simulink model "FSK_switched"  (R2019a)
settings: Solver=ode45  StartTime=0.0  StopTime=10.0  RelTol=1e-3  EnableMultiTasking=on
libraries: commnoisgen2 x1, dspobslib x1
settings Model: Creator=carlos  LastModifiedBy=carlos
settings DataIOCC: LimitDataPoints=on  SaveFormat=Array  SignalLoggingSaveFormat=ModelDataLogs  ReturnWorkspaceOutputs=off
settings OptimizationCC: ExpressionDepthLimit=2147483647  LifeSpan=inf
settings DebuggingCC: UnderspecifiedInitializationDetection=Classic  MergeDetectMultiDrivingBlocksExec=none  SolverPrmCheckMsg=warning  FcnCallInpInsideContextMsg=warning  StateNameClashWarn=warning  SFUnexpectedBacktrackingDiag=warning  SFNoUnconditionalDefaultTransitionDiag=warning  SFExecutionAtInitializationDiag=none  ArithmeticOperatorsInVariantConditions=warning
settings HardwareCC: ProdBitPerPointer=32  ProdBitPerSizeT=32  ProdBitPerPtrDiffT=32  ProdLargestAtomicFloat=None  ProdIntDivRoundTo=Undefined  ProdEndianess=Unspecified  ProdWordSize=32  ProdHWDeviceType=32-bit Generic
settings ModelReferenceCC: PropagateSignalLabelsOutOfModel=off
settings SFSimCC: SimUseLocalCustomCode=off
settings RTWCC: RTWUseLocalCustomCode=off
settings CodeAppCC: StateflowObjectComments=on
settings GRTTargetCC: TargetLangStandard=C89/C90 (ANSI)  CombineOutputUpdateFcns=off  GRTInterface=on
settings ConfigComp: CovMetricSettings=dw  CovHtmlReporting=on  CovSaveCumulativeToWorkspaceVar=on  CovSaveSingleToWorkspaceVar=on  CovExternalEMLEnable=off

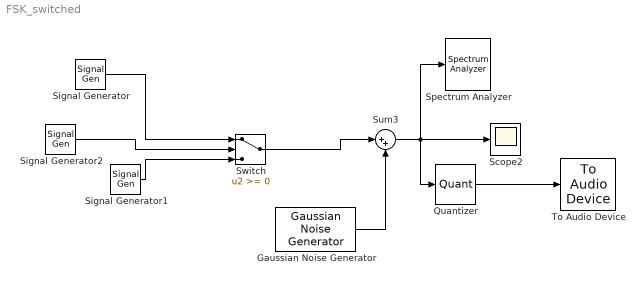
== system FSK_switched ==
  Gaussian Noise Generator : commnoisgen2/Gaussian Noise Generator  m=0  d=0  s=200  Ts=1e-4  frameBased=off  sampPerFrame=1  orient=off  outDataType=double
      settings: SourceProductName=Communications Toolbox  SourceProductBaseCode=CM
  Quantizer : Quantizer  QuantizationInterval=0.01  LinearizeAsGain=off  SampleTime=1/44100
  Scope2 : Scope
  Signal Generator : SignalGenerator  Amplitude=0.5  Frequency=1500
  Signal Generator1 : SignalGenerator  Amplitude=0.5  Frequency=800
  Signal Generator2 : SignalGenerator  WaveForm=square  Amplitude=0.5  Frequency=3
  Spectrum Analyzer : SpectrumAnalyzer
  Sum3 : Sum  Inputs=|++  SampleTime=1e-4
  Switch : Switch
  To Audio Device : dspobslib/To Audio Device  deviceName=Default  inheritSampleRate=off  sampleRate=44100  deviceDatatype=Determine from input data type  autoBufferSize=on  bufferSize=4096  queueDuration=1.0  defaultOutputChannelMapping=on  outputChannelMapping=1:2  outputNumUnderrunSamples=off
      settings: SourceProductName=DSP System Toolbox  SourceProductBaseCode=DS
  wires:
  Signal Generator/1 -> Switch/1
  Signal Generator1/1 -> Switch/3
  Signal Generator2/1 -> Switch/2
  Gaussian Noise Generator/1 -> Sum3/2
  Switch/1 -> Sum3/1
  Quantizer/1 -> To Audio Device/1
  Sum3/1 -> Spectrum Analyzer/1, Scope2/1, Quantizer/1
